simulink model "cont_dis_regler"  (Simulink 7.3)
settings: Solver=ode45  StartTime=0.0  StopTime=10  RelTol=1e-3
values from neighbouring files (symbols this model uses):
  a_0 = T_1/T_2*exp(-T_a*(1/T_2-1/T_1))    [koeff.m]
  a_1 = T_1/T_2*exp(-T_a/T_2)    [koeff.m]
  b_1 = exp(-T_a/T_2)    [koeff.m]
undefined symbols (not defined in the file or in its folder): k, T_1, T_2, T_w, x_c
settings Model: Creator=akoerner  LastModifiedBy=akoerner
settings DebuggingCC: SaveWithParameterizedLinksMsg=none

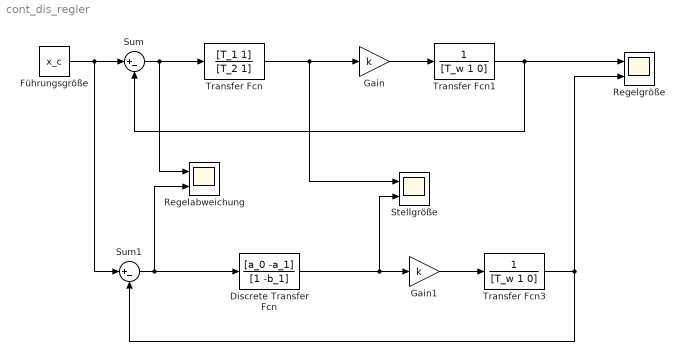
== system cont_dis_regler ==
  Discrete Transfer Fcn : DiscreteTransferFcn  Numerator=[a_0 -a_1]  Denominator=[1 -b_1]
  Führungsgröße : Constant  Value=x_c  OutDataType=fixdt(1, 16)  OutScaling=2^0
  Gain : Gain  Gain=k  ParameterDataType=fixdt(1, 16)  ParameterScaling=2^0  OutDataType=fixdt(1, 16)  OutScaling=2^0
  Gain1 : Gain  Gain=k  ParameterDataType=fixdt(1, 16)  ParameterScaling=2^0  OutDataType=fixdt(1, 16)  OutScaling=2^0
  Regelabweichung : Scope  NumInputPorts=2
      settings: YMin=-5~-5  YMax=5~5  SaveName=ScopeData2
  Regelgröße : Scope  NumInputPorts=2
      settings: YMin=-5~-5  YMax=5~5
  Stellgröße : Scope  NumInputPorts=2
      settings: YMin=-5~-5  YMax=5~5  SaveName=ScopeData3
  Sum : Sum  Inputs=|+-  OutDataType=fixdt(1, 16)  OutScaling=2^0
  Sum1 : Sum  Inputs=|+-  OutDataType=fixdt(1, 16)  OutScaling=2^0
  Transfer Fcn : TransferFcn  Numerator=[T_1 1]  Denominator=[T_2 1]
  Transfer Fcn1 : TransferFcn  Denominator=[T_w 1 0]
  Transfer Fcn3 : TransferFcn  Denominator=[T_w 1 0]
  wires:
  Sum/1 -> Transfer Fcn/1, Regelabweichung/1
  Transfer Fcn/1 -> Gain/1, Stellgröße/1
  Gain/1 -> Transfer Fcn1/1
  Transfer Fcn1/1 -> Regelgröße/1, Sum/2
  Führungsgröße/1 -> Sum/1, Sum1/1
  Gain1/1 -> Transfer Fcn3/1
  Transfer Fcn3/1 -> Sum1/2, Regelgröße/2
  Discrete Transfer Fcn/1 -> Gain1/1, Stellgröße/2
  Sum1/1 -> Regelabweichung/2, Discrete Transfer Fcn/1
